simulink model "ENV"  (R2024b)
settings: Solver=FixedStepDiscrete  StartTime=0.0  StopTime=1  FixedStep=0.001  RelTol=1e-3  EnableMultiTasking=on
PreLoadFcn:
  | load('CAN_MESSAGE_bus.mat');
libraries: stm32blockslib x62, canmsglib x28, simulink x6, stm32f4xxblockslib x3
(part 2 of 5)

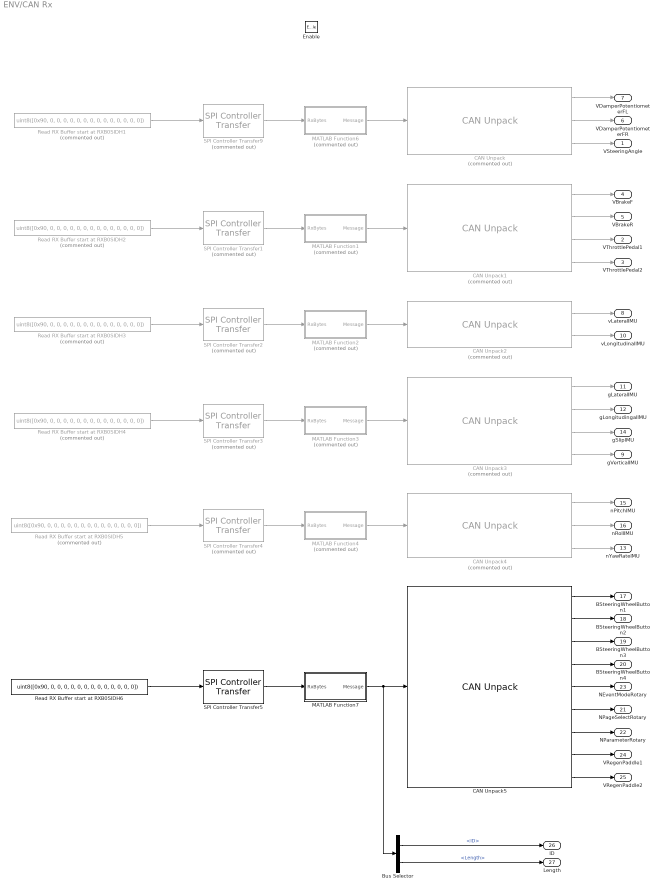
== system ENV/CAN Rx ==
  Enable : EnablePort
  Bus Selector : BusSelector  OutputSignals=ID,Length
  CAN Unpack : canmsglib/CAN Unpack  Commented=on  CANdbFile=C:\Users\oxbro\Documents\STM32CustomProjects\VCUSTM32\OBR26_Controls_30-7-26\CAN\CAN3\CAN3_03.08.26.dbc  MsgList=DDU7_SteerDamper  MsgName=DDU7_SteerDamper  MsgIDType=Standard (11-bit identifier)  MsgIdentifier=257  MsgLength=8  SignalInfo={'VDamperPotentiometerFL','16','13','LE','unsigned','Standard','0','1','0','0','8191';'VDamperPotentiometerFR','29','13','LE','unsigned','Standard','0','1','0','0','8191';'VSteeringAngle','0','13','LE','unsigned','Standard','0','1','0','0','8191'}  IDPort=off  TimestampPort=off  ErrorPort=off  RemotePort=off  LengthPort=off  StatusPort=off  ApplyMinMax=off
      settings: LibrarySourceBlock=stmutilitieslib/CAN Unpack  DataFormat=CANdb specified signals
  CAN Unpack1 : canmsglib/CAN Unpack  Commented=on  CANdbFile=C:\Users\oxbro\Documents\STM32CustomProjects\VCUSTM32\OBR26_Controls_30-7-26\CAN\CAN3\CAN3_03.08.26.dbc  MsgList=DDU7_ThrBrake  MsgName=DDU7_ThrBrake  MsgIDType=Standard (11-bit identifier)  MsgIdentifier=256  MsgLength=8  SignalInfo={'VBrakeF','0','16','LE','unsigned','Standard','0','1','0','0','3276.75';'VBrakeR','16','16','LE','unsigned','Standard','0','1','0','0','65535';'VThrottlePedal1','32','16','LE','unsigned','Standard','0','1','0','0','65535';'VThrottlePedal2','48','16','LE','unsigned','Standard','0','1','0','0','65535'}  IDPort=off  TimestampPort=off  ErrorPort=off  RemotePort=off  LengthPort=off  StatusPort=off  ApplyMinMax=off
      settings: LibrarySourceBlock=stmutilitieslib/CAN Unpack  DataFormat=CANdb specified signals
  CAN Unpack2 : canmsglib/CAN Unpack  Commented=on  CANdbFile=C:\Users\oxbro\Documents\STM32CustomProjects\VCUSTM32\OBR26_Controls_30-7-26\CAN\CAN3\CAN3_03.08.26.dbc  MsgList=IMU_0x604  MsgName=IMU_0x604  MsgIDType=Standard (11-bit identifier)  MsgIdentifier=1540  MsgLength=8  SignalInfo={'vLateralIMU','16','16','LE','signed','Standard','0','0.01','0','-327.68','327.67';'vLongitudinalIMU','0','16','LE','signed','Standard','0','0.01','0','-327.68','327.67'}  IDPort=off  TimestampPort=off  ErrorPort=off  RemotePort=off  LengthPort=off  StatusPort=off  ApplyMinMax=off
      settings: LibrarySourceBlock=stmutilitieslib/CAN Unpack  DataFormat=CANdb specified signals
  CAN Unpack3 : canmsglib/CAN Unpack  Commented=on  CANdbFile=C:\Users\oxbro\Documents\STM32CustomProjects\VCUSTM32\OBR26_Controls_30-7-26\CAN\CAN3\CAN3_03.08.26.dbc  MsgList=IMU_0x606  MsgName=IMU_0x606  MsgIDType=Standard (11-bit identifier)  MsgIdentifier=1542  MsgLength=8  SignalInfo={'gLateralIMU','16','16','LE','signed','Standard','0','0.01','0','-327.68','327.67';'gLongitudinalIMU','0','16','LE','signed','Standard','0','0.01','0','-327.68','327.67';'gSlipIMU','48','16','LE','signed','Standard','0','0.01','0','-327.68','327.67';'gVerticalIMU','32','16','LE','signed','Standard','0','0.01','0','-327.68','327.67'}  IDPort=off  TimestampPort=off  ErrorPort=off  RemotePort=off  LengthPort=off  StatusPort=off  ApplyMinMax=off
      settings: LibrarySourceBlock=stmutilitieslib/CAN Unpack  DataFormat=CANdb specified signals
  CAN Unpack4 : canmsglib/CAN Unpack  Commented=on  CANdbFile=C:\Users\oxbro\Documents\STM32CustomProjects\VCUSTM32\OBR26_Controls_30-7-26\CAN\CAN3\CAN3_03.08.26.dbc  MsgList=IMU_0x609  MsgName=IMU_0x609  MsgIDType=Standard (11-bit identifier)  MsgIdentifier=1545  MsgLength=8  SignalInfo={'nPitchIMU','16','16','LE','signed','Standard','0','0.01','0','-327.68','327.67';'nRollIMU','0','16','LE','signed','Standard','0','0.01','0','-327.68','327.67';'nYawRateIMU','32','16','LE','signed','Standard','0','0.01','0','-327.68','327.67'}  IDPort=off  TimestampPort=off  ErrorPort=off  RemotePort=off  LengthPort=off  StatusPort=off  ApplyMinMax=off
      settings: LibrarySourceBlock=stmutilitieslib/CAN Unpack  DataFormat=CANdb specified signals
  CAN Unpack5 : canmsglib/CAN Unpack  CANdbFile=C:\Users\oxbro\Documents\STM32CustomProjects\VCUSTM32\OBR26_Controls_30-7-26\CAN\CAN3\CAN3_03.08.26.dbc  MsgList=STW_0x1FB  MsgName=STW_0x1FB  MsgIDType=Standard (11-bit identifier)  MsgIdentifier=507  MsgLength=6  SignalInfo={'BSteeringWheelButton1','0','1','LE','unsigned','Standard','0','1','0','0','1';'BSteeringWheelButton2','1','1','LE','unsigned','Standard','0','1','0','0','1';'BSteeringWheelButton3','2','1','LE','unsigned','Standard','0','1','0','0','1';'BSteeringWheelButton4','3','1','LE','unsigned','Standard','0','1','0','0','1';'NEventModeRotary','20','8','LE','unsigned','Standard','0','1','1','1','16';'NPageSelectRotary','4','8','LE','unsigned','Standard','0','1','1','1','16';'NParameterRotary','12','8','LE','unsigned','Standard','0','1','1','1','16';'VRegenPaddle1','28','8','LE','unsigned','Standard','0','0.0129','0','0','3.2895';'VRegenPaddle2','36','8','LE','unsigned','Standard','0','0.0129','0','0','3.2895'}  IDPort=off  TimestampPort=off  ErrorPort=off  RemotePort=off  LengthPort=off  StatusPort=off  ApplyMinMax=off
      settings: LibrarySourceBlock=stmutilitieslib/CAN Unpack  DataFormat=CANdb specified signals
  MATLAB Function1 : MATLAB Function  Commented=on  TreatAsAtomicUnit=on
  MATLAB Function2 : MATLAB Function  Commented=on  TreatAsAtomicUnit=on
  MATLAB Function3 : MATLAB Function  Commented=on  TreatAsAtomicUnit=on
  MATLAB Function4 : MATLAB Function  Commented=on  TreatAsAtomicUnit=on
  MATLAB Function6 : MATLAB Function  Commented=on  TreatAsAtomicUnit=on
  MATLAB Function7 : MATLAB Function  TreatAsAtomicUnit=on
  Read RX Buffer start at RXB0SIDH{1..5} (5 alike) : Constant  Commented=on  Value=uint8([0x90, 0, 0, 0, 0, 0, 0, 0, 0, 0, 0, 0, 0, 0, 0])
  Read RX Buffer start at RXB0SIDH6 : Constant  Value=uint8([0x90, 0, 0, 0, 0, 0, 0, 0, 0, 0, 0, 0, 0, 0])
  SPI Controller Transfer1 : stm32blockslib/SPI Controller Transfer  Priority=2  Commented=on  SPIModuleSelect=SPI1  ClockPolarity=Low  ClockPhase=1 Edge  SPIModule=uint32(0)  Mode=Master  BusSpeed=uint32(1000000)  FirstBitToTransfer=Most significant bit (MSB)  ClockMode=0  BlockFunction=Transfer  EnableRegisterAddress=off  RegisterAddress=0  OutputDataType=uint8  OutputDataLength=1  OutputStatus=off  BlockingMode=on  Timeout=0.01  DataBits=8  UseCustomSSPin=Explicit GPIO calls  ActiveLowSSPin=Active low  Port_Select=GPIOA  Pin=1
      settings: LibrarySourceBlock=stm32h7xxblockslib/SPI Controller Transfer
  SPI Controller Transfer2 : stm32blockslib/SPI Controller Transfer  Priority=3  Commented=on  SPIModuleSelect=SPI1  ClockPolarity=Low  ClockPhase=1 Edge  SPIModule=uint32(0)  Mode=Master  BusSpeed=uint32(1000000)  FirstBitToTransfer=Most significant bit (MSB)  ClockMode=0  BlockFunction=Transfer  EnableRegisterAddress=off  RegisterAddress=0  OutputDataType=uint8  OutputDataLength=1  OutputStatus=off  BlockingMode=on  Timeout=0.01  DataBits=8  UseCustomSSPin=Explicit GPIO calls  ActiveLowSSPin=Active low  Port_Select=GPIOA  Pin=1
      settings: LibrarySourceBlock=stm32h7xxblockslib/SPI Controller Transfer
  SPI Controller Transfer3 : stm32blockslib/SPI Controller Transfer  Priority=4  Commented=on  SPIModuleSelect=SPI1  ClockPolarity=Low  ClockPhase=1 Edge  SPIModule=uint32(0)  Mode=Master  BusSpeed=uint32(1000000)  FirstBitToTransfer=Most significant bit (MSB)  ClockMode=0  BlockFunction=Transfer  EnableRegisterAddress=off  RegisterAddress=0  OutputDataType=uint8  OutputDataLength=1  OutputStatus=off  BlockingMode=on  Timeout=0.01  DataBits=8  UseCustomSSPin=Explicit GPIO calls  ActiveLowSSPin=Active low  Port_Select=GPIOA  Pin=1
      settings: LibrarySourceBlock=stm32h7xxblockslib/SPI Controller Transfer
  SPI Controller Transfer4 : stm32blockslib/SPI Controller Transfer  Priority=5  Commented=on  SPIModuleSelect=SPI1  ClockPolarity=Low  ClockPhase=1 Edge  SPIModule=uint32(0)  Mode=Master  BusSpeed=uint32(1000000)  FirstBitToTransfer=Most significant bit (MSB)  ClockMode=0  BlockFunction=Transfer  EnableRegisterAddress=off  RegisterAddress=0  OutputDataType=uint8  OutputDataLength=1  OutputStatus=off  BlockingMode=on  Timeout=0.01  DataBits=8  UseCustomSSPin=Explicit GPIO calls  ActiveLowSSPin=Active low  Port_Select=GPIOA  Pin=1
      settings: LibrarySourceBlock=stm32h7xxblockslib/SPI Controller Transfer
  SPI Controller Transfer5 : stm32blockslib/SPI Controller Transfer  Priority=6  SPIModuleSelect=SPI1  ClockPolarity=Low  ClockPhase=1 Edge  SPIModule=uint32(0)  Mode=Master  BusSpeed=uint32(1000000)  FirstBitToTransfer=Most significant bit (MSB)  ClockMode=0  BlockFunction=Transfer  EnableRegisterAddress=off  RegisterAddress=0  OutputDataType=uint8  OutputDataLength=1  OutputStatus=off  BlockingMode=on  Timeout=0.01  DataBits=8  UseCustomSSPin=Explicit GPIO calls  ActiveLowSSPin=Active low  Port_Select=GPIOA  Pin=1
      settings: LibrarySourceBlock=stm32h7xxblockslib/SPI Controller Transfer
  SPI Controller Transfer9 : stm32blockslib/SPI Controller Transfer  Priority=1  Commented=on  SPIModuleSelect=SPI1  ClockPolarity=Low  ClockPhase=1 Edge  SPIModule=uint32(0)  Mode=Master  BusSpeed=uint32(1000000)  FirstBitToTransfer=Most significant bit (MSB)  ClockMode=0  BlockFunction=Transfer  EnableRegisterAddress=off  RegisterAddress=0  OutputDataType=uint8  OutputDataLength=1  OutputStatus=off  BlockingMode=on  Timeout=0.01  DataBits=8  UseCustomSSPin=Explicit GPIO calls  ActiveLowSSPin=Active low  Port_Select=GPIOA  Pin=1
      settings: LibrarySourceBlock=stm32h7xxblockslib/SPI Controller Transfer
  VSteeringAngle : Outport  OutDataTypeStr=double
  VThrottlePedal1 : Outport  Port=2  OutDataTypeStr=double
  VThrottlePedal2 : Outport  Port=3  OutDataTypeStr=double
  VBrakeF : Outport  Port=4  OutDataTypeStr=double
  VBrakeR : Outport  Port=5  OutDataTypeStr=double
  VDamperPotentiometerFR : Outport  Port=6  OutDataTypeStr=double
  VDamperPotentiometerFL : Outport  Port=7  OutDataTypeStr=double
  vLateralIMU : Outport  Port=8  OutDataTypeStr=double
  gVerticalIMU : Outport  Port=9  OutDataTypeStr=double
  vLongitudinalIMU : Outport  Port=10  OutDataTypeStr=double
  gLateralIMU : Outport  Port=11  OutDataTypeStr=double
  gLongitudingalIMU : Outport  Port=12  OutDataTypeStr=double
  nYawRateIMU : Outport  Port=13  OutDataTypeStr=double
  gSlipIMU : Outport  Port=14  OutDataTypeStr=double
  nPitchIMU : Outport  Port=15  OutDataTypeStr=double
  nRollIMU : Outport  Port=16  OutDataTypeStr=double
  BSteeringWheelButton1 : Outport  Port=17  OutDataTypeStr=boolean
  BSteeringWheelButton2 : Outport  Port=18  OutDataTypeStr=boolean
  BSteeringWheelButton3 : Outport  Port=19  OutDataTypeStr=boolean
  BSteeringWheelButton4 : Outport  Port=20  OutDataTypeStr=boolean
  NPageSelectRotary : Outport  Port=21  OutDataTypeStr=double
  NParameterRotary : Outport  Port=22  OutDataTypeStr=double
  NEventModeRotary : Outport  Port=23  OutDataTypeStr=double
  VRegenPaddle1 : Outport  Port=24  OutDataTypeStr=double
  VRegenPaddle2 : Outport  Port=25  OutDataTypeStr=double
  ID : Outport  Port=26
  Length : Outport  Port=27
  wires:
  CAN Unpack/1 -> VDamperPotentiometerFL/1
  CAN Unpack/2 -> VDamperPotentiometerFR/1
  CAN Unpack1/2 -> VBrakeR/1
  CAN Unpack1/1 -> VBrakeF/1
  CAN Unpack1/3 -> VThrottlePedal1/1
  CAN Unpack1/4 -> VThrottlePedal2/1
  CAN Unpack/3 -> VSteeringAngle/1
  SPI Controller Transfer9/1 -> MATLAB Function6/1(RxBytes)
  MATLAB Function6/1(Message) -> CAN Unpack/1
  MATLAB Function1/1(Message) -> CAN Unpack1/1
  SPI Controller Transfer1/1 -> MATLAB Function1/1(RxBytes)
  SPI Controller Transfer2/1 -> MATLAB Function2/1(RxBytes)
  MATLAB Function2/1(Message) -> CAN Unpack2/1
  CAN Unpack2/2 -> vLongitudinalIMU/1
  CAN Unpack2/1 -> vLateralIMU/1
  MATLAB Function3/1(Message) -> CAN Unpack3/1
  SPI Controller Transfer3/1 -> MATLAB Function3/1(RxBytes)
  CAN Unpack3/4 -> gVerticalIMU/1
  CAN Unpack3/3 -> gSlipIMU/1
  CAN Unpack3/2 -> gLongitudingalIMU/1
  CAN Unpack3/1 -> gLateralIMU/1
  CAN Unpack4/2 -> nRollIMU/1
  CAN Unpack4/3 -> nYawRateIMU/1
  CAN Unpack4/1 -> nPitchIMU/1
  SPI Controller Transfer4/1 -> MATLAB Function4/1(RxBytes)
  MATLAB Function4/1(Message) -> CAN Unpack4/1
  SPI Controller Transfer5/1 -> MATLAB Function7/1(RxBytes)
  CAN Unpack5/2 -> BSteeringWheelButton2/1
  CAN Unpack5/1 -> BSteeringWheelButton1/1
  CAN Unpack5/3 -> BSteeringWheelButton3/1
  CAN Unpack5/4 -> BSteeringWheelButton4/1
  CAN Unpack5/9 -> VRegenPaddle2/1
  CAN Unpack5/8 -> VRegenPaddle1/1
  CAN Unpack5/7 -> NParameterRotary/1
  CAN Unpack5/6 -> NPageSelectRotary/1
  CAN Unpack5/5 -> NEventModeRotary/1
  Read RX Buffer start at RXB0SIDH1/1 -> SPI Controller Transfer9/1
  Read RX Buffer start at RXB0SIDH6/1 -> SPI Controller Transfer5/1
  Read RX Buffer start at RXB0SIDH5/1 -> SPI Controller Transfer4/1
  Read RX Buffer start at RXB0SIDH4/1 -> SPI Controller Transfer3/1
  Read RX Buffer start at RXB0SIDH3/1 -> SPI Controller Transfer2/1
  Read RX Buffer start at RXB0SIDH2/1 -> SPI Controller Transfer1/1
  MATLAB Function7/1(Message) -> Bus Selector/1, CAN Unpack5/1
  Bus Selector/2 -> Length/1  "<Length>"
  Bus Selector/1 -> ID/1  "<ID>"

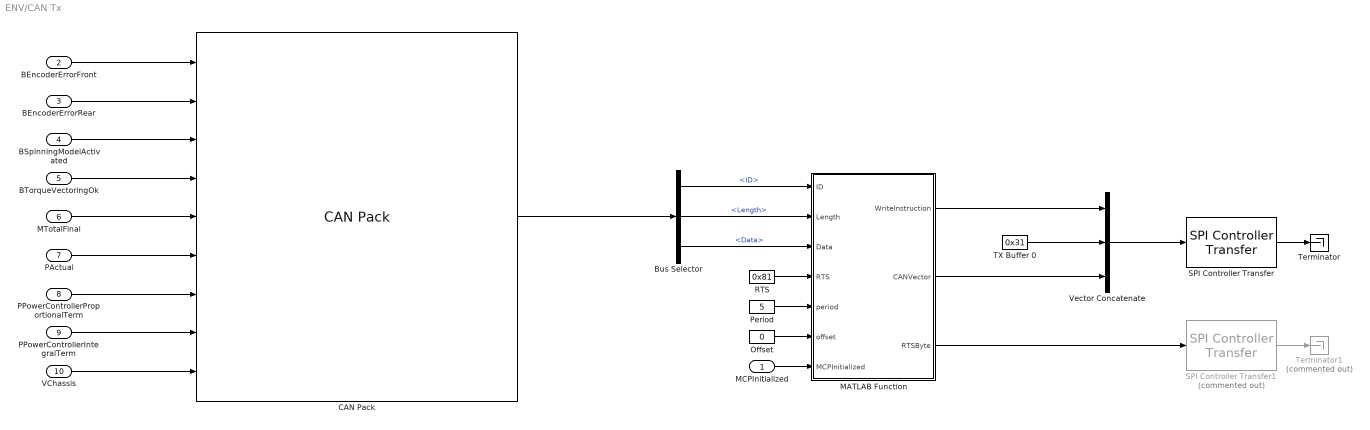
== system ENV/CAN Tx ==
  MCPInitialized : Inport
  BEncoderErrorFront : Inport  Port=2
  BEncoderErrorRear : Inport  Port=3
  BSpinningModelActivated : Inport  Port=4
  BTorqueVectoringOk : Inport  Port=5
  MTotalFinal : Inport  Port=6
  PActual : Inport  Port=7
  PPowerControllerProportionalTerm : Inport  Port=8
  PPowerControllerIntegralTerm : Inport  Port=9
  VChassis : Inport  Port=10
  Bus Selector : BusSelector  OutputSignals=ID,Length,Data
  CAN Pack : canmsglib/CAN Pack  CANdbFile=C:\Users\William\Downloads\VCUSTM32\BaselineControls\CAN\CAN3_baseline.dbc  MsgList=(none)  MsgName=Etas_Signals_01  MsgIDType=Standard (11-bit identifier)  MsgIdentifier=2022  CANIDInput=off  MsgLength=8  Remote=off  ApplyMinMax=off  BusOutput=on  SignalInfo={'BEncoderErrorFront','62','1','LE','unsigned','Standard','0','1','0','0','1';'BEncoderErrorRear','63','1','LE','unsigned','Standard','0','1','0','0','1';'BSpinningModelActivated','60','1','LE','unsigned','Standard','0','1','0','0','1';'BTorqueVectoringOk','61','1','LE','unsigned','Standard','0','1','0','0','1';'MTotalFinal','11','14','LE','signed','Standard','0','0.1','300','-Inf','Inf';'PActual','25','14','LE','signed','Standard','0','0.01','30','-51.92','111.91';'PPowerControlerProportionalTerm','0','11','LE','signed','Standard','0','0.01','0','-10.24','10.23';'PPowerControllerIntergralTerm','49','11','LE','signed','Standard','0','0.01','0','-10.24','10.23';'vChassis','39','10','LE','signed','Standard','0','0.1','0','-51.2','51.1'}
      settings: LibrarySourceBlock=stmutilitieslib/CAN Pack  DataFormat=CANdb specified signals
  MATLAB Function : MATLAB Function  TreatAsAtomicUnit=on
  Offset : Constant  Value=0  OutDataTypeStr=uint16  SampleTime=-1
  Period : Constant  Value=5  OutDataTypeStr=uint16  SampleTime=-1
  RTS : Constant  Value=0x81  OutDataTypeStr=uint8  SampleTime=-1
  SPI Controller Transfer : stm32blockslib/SPI Controller Transfer  Priority=1  SPIModuleSelect=SPI1  ClockPolarity=Low  ClockPhase=1 Edge  SPIModule=uint32(0)  Mode=Master  BusSpeed=uint32(1000000)  FirstBitToTransfer=Most significant bit (MSB)  ClockMode=0  BlockFunction=Transfer  EnableRegisterAddress=off  RegisterAddress=0  OutputDataType=uint8  OutputDataLength=1  OutputStatus=off  BlockingMode=off  Timeout=0.01  DataBits=8  UseCustomSSPin=Explicit GPIO calls  ActiveLowSSPin=Active low  Port_Select=GPIOA  Pin=4
      settings: LibrarySourceBlock=stm32h7xxblockslib/SPI Controller Transfer
  SPI Controller Transfer1 : stm32blockslib/SPI Controller Transfer  Priority=2  Commented=on  SPIModuleSelect=SPI1  ClockPolarity=Low  ClockPhase=1 Edge  SPIModule=uint32(0)  Mode=Master  BusSpeed=uint32(1000000)  FirstBitToTransfer=Most significant bit (MSB)  ClockMode=0  BlockFunction=Transfer  EnableRegisterAddress=off  RegisterAddress=0  OutputDataType=uint8  OutputDataLength=1  OutputStatus=off  BlockingMode=off  Timeout=0.01  DataBits=8  UseCustomSSPin=Explicit GPIO calls  ActiveLowSSPin=Active low  Port_Select=GPIOA  Pin=4
      settings: LibrarySourceBlock=stm32h7xxblockslib/SPI Controller Transfer
  TX Buffer 0 : Constant  Value=0x31  OutDataTypeStr=uint8  SampleTime=-1
  Terminator : Terminator
  Terminator1 : Terminator  Commented=on
  Vector Concatenate : Concatenate  NumInputs=3
  wires:
  CAN Pack/1 -> Bus Selector/1
  BEncoderErrorFront/1 -> CAN Pack/1
  BTorqueVectoringOk/1 -> CAN Pack/4
  BSpinningModelActivated/1 -> CAN Pack/3
  BEncoderErrorRear/1 -> CAN Pack/2
  MTotalFinal/1 -> CAN Pack/5
  PActual/1 -> CAN Pack/6
  PPowerControllerProportionalTerm/1 -> CAN Pack/7
  PPowerControllerIntegralTerm/1 -> CAN Pack/8
  VChassis/1 -> CAN Pack/9
  RTS/1 -> MATLAB Function/4(RTS)
  Bus Selector/1 -> MATLAB Function/1(ID)  "<ID>"
  Bus Selector/2 -> MATLAB Function/2(Length)  "<Length>"
  Bus Selector/3 -> MATLAB Function/3(Data)  "<Data>"
  Offset/1 -> MATLAB Function/6(offset)
  Period/1 -> MATLAB Function/5(period)
  MCPInitialized/1 -> MATLAB Function/7(MCPInitialized)
  Vector Concatenate/1 -> SPI Controller Transfer/1
  MATLAB Function/1(WriteInstruction) -> Vector Concatenate/1
  SPI Controller Transfer1/1 -> Terminator1/1
  TX Buffer 0/1 -> Vector Concatenate/2
  SPI Controller Transfer/1 -> Terminator/1
  MATLAB Function/3(RTSByte) -> SPI Controller Transfer1/1
  MATLAB Function/2(CANVector) -> Vector Concatenate/3

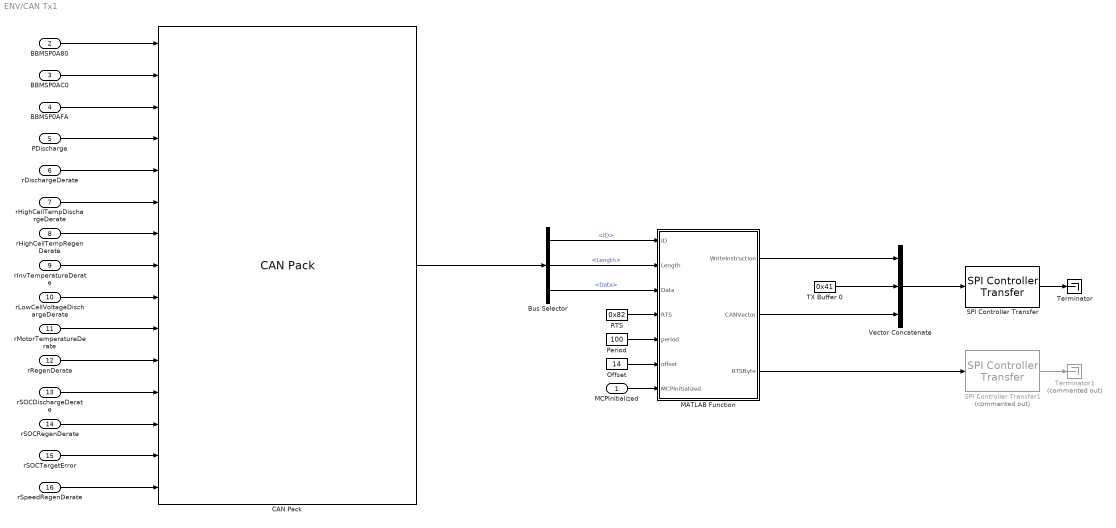
== system ENV/CAN Tx1 ==
  MCPInitialized : Inport
  BBMSP0A80 : Inport  Port=2
  BBMSP0AC0 : Inport  Port=3
  BBMSP0AFA : Inport  Port=4
  PDischarge : Inport  Port=5
  rDischargeDerate : Inport  Port=6
  rHighCellTempDischargeDerate : Inport  Port=7
  rHighCellTempRegenDerate : Inport  Port=8
  rInvTemperatureDerate : Inport  Port=9
  rLowCellVoltageDischargeDerate : Inport  Port=10
  rMotorTemperatureDerate : Inport  Port=11
  rRegenDerate : Inport  Port=12
  rSOCDischargeDerate : Inport  Port=13
  rSOCRegenDerate : Inport  Port=14
  rSOCTargetError : Inport  Port=15
  rSpeedRegenDerate : Inport  Port=16
  Bus Selector : BusSelector  OutputSignals=ID,Length,Data
  CAN Pack : canmsglib/CAN Pack  CANdbFile=C:\Users\William\Downloads\VCUSTM32\BaselineControls\CAN\CAN3_baseline.dbc  MsgList=(none)  MsgName=Etas_Signals_02  MsgIDType=Standard (11-bit identifier)  MsgIdentifier=2023  CANIDInput=off  MsgLength=8  Remote=off  ApplyMinMax=off  BusOutput=on  SignalInfo={'BBMSP0A80','0','1','LE','unsigned','Standard','0','1','0','0','1';'BBMSP0AC0','1','1','LE','unsigned','Standard','0','1','0','0','1';'BBMSP0AFA','2','1','LE','unsigned','Standard','0','1','0','0','1';'PDischarge','43','8','LE','unsigned','Standard','0','1','0','0','255';'rDischargeDerate','35','4','LE','unsigned','Standard','0','0.1','0','0','1.5';'rHighCellTempDischargeDerate','3','4','LE','unsigned','Standard','0','0.1','0','0','1.5';'rHighCellTempRegenDerate','7','4','LE','unsigned','Standard','0','0.1','0','0','1.5';'rInvTemperatureDerate','11','4','LE','unsigned','Standard','0','0.1','0','0','1.5';'rLowCellVoltageDischargeDerate','19','4','LE','unsigned','Standard','0','0.1','0','0','1.5';'rMotorTemperatureDerate','15','4','LE','unsigned','Standard','0','0.1','0','0','1.5';'rRegenDerate','39','4','LE','unsigned','Standard','0','0.1','0','0','1.5';'rSOCDischargeDerate','23','4','LE','unsigned','Standard','0','0.1','0','0','1.5';'rSOCRegenDerate','27','4','LE','unsigned','Standard','0','0.1','0','0','1.5';'rSOCTargetError','51','13','LE','signed','Standard','0','0.001','0','-4.096','4.095';'rSpeedRegenDerate','31','4','LE','unsigned','Standard','0','0.1','0','0','1.5'}
      settings: LibrarySourceBlock=stmutilitieslib/CAN Pack  DataFormat=CANdb specified signals
  MATLAB Function : MATLAB Function  TreatAsAtomicUnit=on
  Offset : Constant  Value=14  OutDataTypeStr=uint16  SampleTime=-1
  Period : Constant  Value=100  OutDataTypeStr=uint16  SampleTime=-1
  RTS : Constant  Value=0x82  OutDataTypeStr=uint8  SampleTime=-1
  SPI Controller Transfer : stm32blockslib/SPI Controller Transfer  Priority=1  SPIModuleSelect=SPI1  ClockPolarity=Low  ClockPhase=1 Edge  SPIModule=uint32(0)  Mode=Master  BusSpeed=uint32(1000000)  FirstBitToTransfer=Most significant bit (MSB)  ClockMode=0  BlockFunction=Transfer  EnableRegisterAddress=off  RegisterAddress=0  OutputDataType=uint8  OutputDataLength=1  OutputStatus=off  BlockingMode=off  Timeout=0.01  DataBits=8  UseCustomSSPin=Explicit GPIO calls  ActiveLowSSPin=Active low  Port_Select=GPIOA  Pin=4
      settings: LibrarySourceBlock=stm32h7xxblockslib/SPI Controller Transfer
  SPI Controller Transfer1 : stm32blockslib/SPI Controller Transfer  Priority=2  Commented=on  SPIModuleSelect=SPI1  ClockPolarity=Low  ClockPhase=1 Edge  SPIModule=uint32(0)  Mode=Master  BusSpeed=uint32(1000000)  FirstBitToTransfer=Most significant bit (MSB)  ClockMode=0  BlockFunction=Transfer  EnableRegisterAddress=off  RegisterAddress=0  OutputDataType=uint8  OutputDataLength=1  OutputStatus=off  BlockingMode=off  Timeout=0.01  DataBits=8  UseCustomSSPin=Explicit GPIO calls  ActiveLowSSPin=Active low  Port_Select=GPIOA  Pin=4
      settings: LibrarySourceBlock=stm32h7xxblockslib/SPI Controller Transfer
  TX Buffer 0 : Constant  Value=0x41  OutDataTypeStr=uint8  SampleTime=-1
  Terminator : Terminator
  Terminator1 : Terminator  Commented=on
  Vector Concatenate : Concatenate  NumInputs=3
  wires:
  BBMSP0AC0/1 -> CAN Pack/2
  BBMSP0A80/1 -> CAN Pack/1
  BBMSP0AFA/1 -> CAN Pack/3
  PDischarge/1 -> CAN Pack/4
  rDischargeDerate/1 -> CAN Pack/5
  rHighCellTempDischargeDerate/1 -> CAN Pack/6
  rHighCellTempRegenDerate/1 -> CAN Pack/7
  rInvTemperatureDerate/1 -> CAN Pack/8
  rLowCellVoltageDischargeDerate/1 -> CAN Pack/9
  rSOCDischargeDerate/1 -> CAN Pack/12
  rSOCRegenDerate/1 -> CAN Pack/13
  rRegenDerate/1 -> CAN Pack/11
  rSOCTargetError/1 -> CAN Pack/14
  rSpeedRegenDerate/1 -> CAN Pack/15
  rMotorTemperatureDerate/1 -> CAN Pack/10
  MATLAB Function/3(RTSByte) -> SPI Controller Transfer1/1
  Bus Selector/3 -> MATLAB Function/3(Data)  "<Data>"
  Offset/1 -> MATLAB Function/6(offset)
  RTS/1 -> MATLAB Function/4(RTS)
  MATLAB Function/1(WriteInstruction) -> Vector Concatenate/1
  Period/1 -> MATLAB Function/5(period)
  Vector Concatenate/1 -> SPI Controller Transfer/1
  Bus Selector/2 -> MATLAB Function/2(Length)  "<Length>"
  SPI Controller Transfer1/1 -> Terminator1/1
  SPI Controller Transfer/1 -> Terminator/1
  TX Buffer 0/1 -> Vector Concatenate/2
  CAN Pack/1 -> Bus Selector/1
  Bus Selector/1 -> MATLAB Function/1(ID)  "<ID>"
  MCPInitialized/1 -> MATLAB Function/7(MCPInitialized)
  MATLAB Function/2(CANVector) -> Vector Concatenate/3

== system ENV/CAN Tx10 ==
  MCPInitialized : Inport
  TEST_NUMBER : Inport  Port=2
  VDamperPotentiometerRL : Inport  Port=3
  VDamperPotentiometerRR : Inport  Port=4
  Bus Selector : BusSelector  OutputSignals=ID,Length,Data
  CAN Pack : canmsglib/CAN Pack  CANdbFile=C:\Users\William\Downloads\VCUSTM32\BaselineControls\CAN\CAN3_baseline.dbc  MsgList=(none)  MsgName=Etas_Signals_11  MsgIDType=Standard (11-bit identifier)  MsgIdentifier=1796  CANIDInput=off  MsgLength=6  Remote=off  ApplyMinMax=off  BusOutput=on  SignalInfo={'TEST_NUMBER','32','16','LE','unsigned','Standard','0','1','0','-32768','32767';'VDamperPotentiometerRL','0','10','LE','unsigned','Standard','0','0.005','0','0','5.115';'VDamperPotentiometerRR','16','10','LE','unsigned','Standard','0','0.005','0','0','5.115'}
      settings: LibrarySourceBlock=stmutilitieslib/CAN Pack  DataFormat=CANdb specified signals
  MATLAB Function : MATLAB Function  TreatAsAtomicUnit=on
  Offset : Constant  Value=8  OutDataTypeStr=uint16  SampleTime=-1
  Period : Constant  Value=100  OutDataTypeStr=uint16  SampleTime=-1
  RTS : Constant  Value=0x82  OutDataTypeStr=uint8  SampleTime=-1
  SPI Controller Transfer : stm32blockslib/SPI Controller Transfer  Priority=1  SPIModuleSelect=SPI1  ClockPolarity=Low  ClockPhase=1 Edge  SPIModule=uint32(0)  Mode=Master  BusSpeed=uint32(1000000)  FirstBitToTransfer=Most significant bit (MSB)  ClockMode=0  BlockFunction=Transfer  EnableRegisterAddress=off  RegisterAddress=0  OutputDataType=uint8  OutputDataLength=1  OutputStatus=off  BlockingMode=off  Timeout=0.01  DataBits=8  UseCustomSSPin=Explicit GPIO calls  ActiveLowSSPin=Active low  Port_Select=GPIOA  Pin=4
      settings: LibrarySourceBlock=stm32h7xxblockslib/SPI Controller Transfer
  SPI Controller Transfer1 : stm32blockslib/SPI Controller Transfer  Priority=2  Commented=on  SPIModuleSelect=SPI1  ClockPolarity=Low  ClockPhase=1 Edge  SPIModule=uint32(0)  Mode=Master  BusSpeed=uint32(1000000)  FirstBitToTransfer=Most significant bit (MSB)  ClockMode=0  BlockFunction=Transfer  EnableRegisterAddress=off  RegisterAddress=0  OutputDataType=uint8  OutputDataLength=1  OutputStatus=off  BlockingMode=off  Timeout=0.01  DataBits=8  UseCustomSSPin=Explicit GPIO calls  ActiveLowSSPin=Active low  Port_Select=GPIOA  Pin=4
      settings: LibrarySourceBlock=stm32h7xxblockslib/SPI Controller Transfer
  TX Buffer 0 : Constant  Value=0x41  OutDataTypeStr=uint8  SampleTime=-1
  Terminator : Terminator
  Terminator1 : Terminator  Commented=on
  Vector Concatenate : Concatenate  NumInputs=3
  wires:
  VDamperPotentiometerRL/1 -> CAN Pack/2
  TEST_NUMBER/1 -> CAN Pack/1
  RTS/1 -> MATLAB Function/4(RTS)
  MATLAB Function/1(WriteInstruction) -> Vector Concatenate/1
  TX Buffer 0/1 -> Vector Concatenate/2
  SPI Controller Transfer1/1 -> Terminator1/1
  MATLAB Function/2(CANVector) -> Vector Concatenate/3
  Offset/1 -> MATLAB Function/6(offset)
  Bus Selector/2 -> MATLAB Function/2(Length)  "<Length>"
  Bus Selector/3 -> MATLAB Function/3(Data)  "<Data>"
  Vector Concatenate/1 -> SPI Controller Transfer/1
  MCPInitialized/1 -> MATLAB Function/7(MCPInitialized)
  Period/1 -> MATLAB Function/5(period)
  Bus Selector/1 -> MATLAB Function/1(ID)  "<ID>"
  CAN Pack/1 -> Bus Selector/1
  SPI Controller Transfer/1 -> Terminator/1
  MATLAB Function/3(RTSByte) -> SPI Controller Transfer1/1
  VDamperPotentiometerRR/1 -> CAN Pack/3

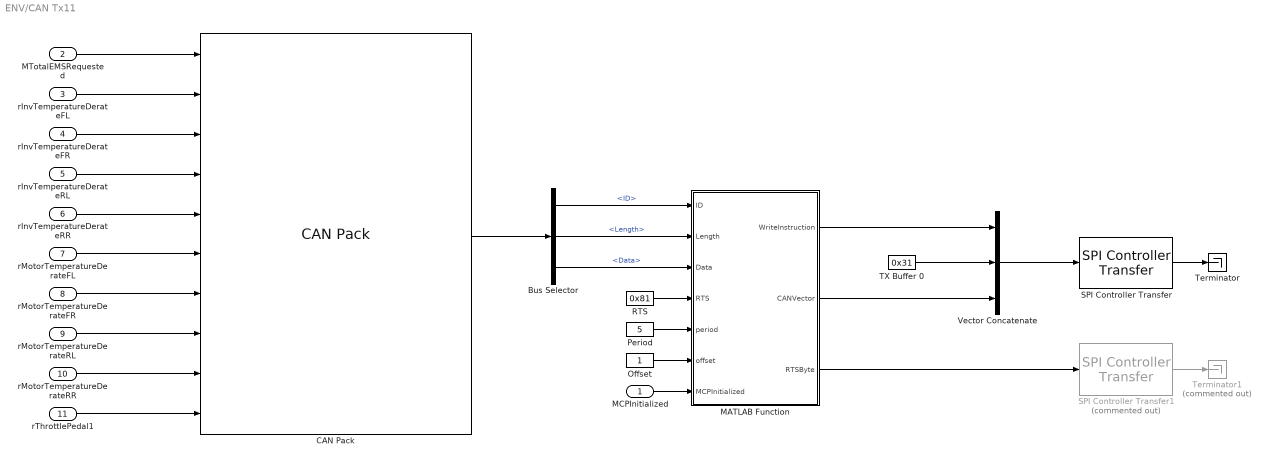
== system ENV/CAN Tx11 ==
  MCPInitialized : Inport
  MTotalEMSRequested : Inport  Port=2
  rInvTemperatureDerateFL : Inport  Port=3
  rInvTemperatureDerateFR : Inport  Port=4
  rInvTemperatureDerateRL : Inport  Port=5
  rInvTemperatureDerateRR : Inport  Port=6
  rMotorTemperatureDerateFL : Inport  Port=7
  rMotorTemperatureDerateFR : Inport  Port=8
  rMotorTemperatureDerateRL : Inport  Port=9
  rMotorTemperatureDerateRR : Inport  Port=10
  rThrottlePedal1 : Inport  Port=11
  Bus Selector : BusSelector  OutputSignals=ID,Length,Data
  CAN Pack : canmsglib/CAN Pack  CANdbFile=C:\Users\William\Downloads\VCUSTM32\BaselineControls\CAN\CAN3_baseline.dbc  MsgList=(none)  MsgName=Etas_Signals_12  MsgIDType=Standard (11-bit identifier)  MsgIdentifier=2039  CANIDInput=off  MsgLength=8  Remote=off  ApplyMinMax=off  BusOutput=on  SignalInfo={'MTotalEMSRequested','32','14','LE','signed','Standard','0','0.1','300','-519.2','1119.1';'rInvTemperatureDerateFL','4','4','LE','unsigned','Standard','0','0.1','0','0','1.5';'rInvTemperatureDerateFR','8','4','LE','unsigned','Standard','0','0.1','0','0','1.5';'rInvTemperatureDerateRL','12','4','LE','unsigned','Standard','0','0.1','0','0','1.5';'rInvTemperatureDerateRR','16','4','LE','unsigned','Standard','0','0.1','0','0','1.5';'rMotorTemperatureDerateFL','20','4','LE','unsigned','Standard','0','0.1','0','0','1.5';'rMotorTemperatureDerateFR','24','4','LE','unsigned','Standard','0','0.1','0','0','1.5';'rMotorTemperatureDerateRL','28','4','LE','unsigned','Standard','0','0.1','0','-Inf','Inf';'rMotorTemperatureDerateRR','0','4','LE','unsigned','Standard','0','0.1','0','0','1.5';'rThrottlePedal1','46','10','LE','unsigned','Standard','0','0.1','0','0','102.3'}
      settings: LibrarySourceBlock=stmutilitieslib/CAN Pack  DataFormat=CANdb specified signals
  MATLAB Function : MATLAB Function  TreatAsAtomicUnit=on
  Offset : Constant  OutDataTypeStr=uint16  SampleTime=-1
  Period : Constant  Value=5  OutDataTypeStr=uint16  SampleTime=-1
  RTS : Constant  Value=0x81  OutDataTypeStr=uint8  SampleTime=-1
  SPI Controller Transfer : stm32blockslib/SPI Controller Transfer  Priority=1  SPIModuleSelect=SPI1  ClockPolarity=Low  ClockPhase=1 Edge  SPIModule=uint32(0)  Mode=Master  BusSpeed=uint32(1000000)  FirstBitToTransfer=Most significant bit (MSB)  ClockMode=0  BlockFunction=Transfer  EnableRegisterAddress=off  RegisterAddress=0  OutputDataType=uint8  OutputDataLength=1  OutputStatus=off  BlockingMode=off  Timeout=0.01  DataBits=8  UseCustomSSPin=Explicit GPIO calls  ActiveLowSSPin=Active low  Port_Select=GPIOA  Pin=4
      settings: LibrarySourceBlock=stm32h7xxblockslib/SPI Controller Transfer
  SPI Controller Transfer1 : stm32blockslib/SPI Controller Transfer  Priority=2  Commented=on  SPIModuleSelect=SPI1  ClockPolarity=Low  ClockPhase=1 Edge  SPIModule=uint32(0)  Mode=Master  BusSpeed=uint32(1000000)  FirstBitToTransfer=Most significant bit (MSB)  ClockMode=0  BlockFunction=Transfer  EnableRegisterAddress=off  RegisterAddress=0  OutputDataType=uint8  OutputDataLength=1  OutputStatus=off  BlockingMode=off  Timeout=0.01  DataBits=8  UseCustomSSPin=Explicit GPIO calls  ActiveLowSSPin=Active low  Port_Select=GPIOA  Pin=4
      settings: LibrarySourceBlock=stm32h7xxblockslib/SPI Controller Transfer
  TX Buffer 0 : Constant  Value=0x31  OutDataTypeStr=uint8  SampleTime=-1
  Terminator : Terminator
  Terminator1 : Terminator  Commented=on
  Vector Concatenate : Concatenate  NumInputs=3
  wires:
  rInvTemperatureDerateFL/1 -> CAN Pack/2
  MTotalEMSRequested/1 -> CAN Pack/1
  rInvTemperatureDerateFR/1 -> CAN Pack/3
  rInvTemperatureDerateRL/1 -> CAN Pack/4
  rInvTemperatureDerateRR/1 -> CAN Pack/5
  rMotorTemperatureDerateFL/1 -> CAN Pack/6
  rMotorTemperatureDerateFR/1 -> CAN Pack/7
  rMotorTemperatureDerateRL/1 -> CAN Pack/8
  rMotorTemperatureDerateRR/1 -> CAN Pack/9
  rThrottlePedal1/1 -> CAN Pack/10
  RTS/1 -> MATLAB Function/4(RTS)
  MATLAB Function/1(WriteInstruction) -> Vector Concatenate/1
  TX Buffer 0/1 -> Vector Concatenate/2
  SPI Controller Transfer1/1 -> Terminator1/1
  MATLAB Function/2(CANVector) -> Vector Concatenate/3
  Offset/1 -> MATLAB Function/6(offset)
  Bus Selector/2 -> MATLAB Function/2(Length)  "<Length>"
  Bus Selector/3 -> MATLAB Function/3(Data)  "<Data>"
  Vector Concatenate/1 -> SPI Controller Transfer/1
  MCPInitialized/1 -> MATLAB Function/7(MCPInitialized)
  Period/1 -> MATLAB Function/5(period)
  Bus Selector/1 -> MATLAB Function/1(ID)  "<ID>"
  CAN Pack/1 -> Bus Selector/1
  SPI Controller Transfer/1 -> Terminator/1
  MATLAB Function/3(RTSByte) -> SPI Controller Transfer1/1

== system ENV/CAN Tx12 ==
  MCPInitialized : Inport
  nMotorFL : Inport  Port=2
  nMotorFR : Inport  Port=3
  nMotorRL : Inport  Port=4
  nMotorRR : Inport  Port=5
  Bus Selector : BusSelector  OutputSignals=ID,Length,Data
  CAN Pack : canmsglib/CAN Pack  CANdbFile=C:\Users\William\Downloads\VCUSTM32\BaselineControls\CAN\CAN3_baseline.dbc  MsgList=(none)  MsgName=Etas_Signals_13  MsgIDType=Standard (11-bit identifier)  MsgIdentifier=2008  CANIDInput=off  MsgLength=8  Remote=off  ApplyMinMax=off  BusOutput=on  SignalInfo={'nMotorFL','0','16','LE','signed','Standard','0','1','0','-32768','32767';'nMotorFR','16','16','LE','signed','Standard','0','1','0','-32768','32767';'nMotorRL','32','16','LE','signed','Standard','0','1','0','-32768','32767';'nMotorRR','48','16','LE','signed','Standard','0','1','0','-32768','32767'}
      settings: LibrarySourceBlock=stmutilitieslib/CAN Pack  DataFormat=CANdb specified signals
  MATLAB Function : MATLAB Function  TreatAsAtomicUnit=on
  Offset : Constant  OutDataTypeStr=uint16  SampleTime=-1
  Period : Constant  Value=10  OutDataTypeStr=uint16  SampleTime=-1
  RTS : Constant  Value=0x82  OutDataTypeStr=uint8  SampleTime=-1
  SPI Controller Transfer : stm32blockslib/SPI Controller Transfer  Priority=1  SPIModuleSelect=SPI1  ClockPolarity=Low  ClockPhase=1 Edge  SPIModule=uint32(0)  Mode=Master  BusSpeed=uint32(1000000)  FirstBitToTransfer=Most significant bit (MSB)  ClockMode=0  BlockFunction=Transfer  EnableRegisterAddress=off  RegisterAddress=0  OutputDataType=uint8  OutputDataLength=1  OutputStatus=off  BlockingMode=off  Timeout=0.01  DataBits=8  UseCustomSSPin=Explicit GPIO calls  ActiveLowSSPin=Active low  Port_Select=GPIOA  Pin=4
      settings: LibrarySourceBlock=stm32h7xxblockslib/SPI Controller Transfer
  SPI Controller Transfer1 : stm32blockslib/SPI Controller Transfer  Priority=2  Commented=on  SPIModuleSelect=SPI1  ClockPolarity=Low  ClockPhase=1 Edge  SPIModule=uint32(0)  Mode=Master  BusSpeed=uint32(1000000)  FirstBitToTransfer=Most significant bit (MSB)  ClockMode=0  BlockFunction=Transfer  EnableRegisterAddress=off  RegisterAddress=0  OutputDataType=uint8  OutputDataLength=1  OutputStatus=off  BlockingMode=off  Timeout=0.01  DataBits=8  UseCustomSSPin=Explicit GPIO calls  ActiveLowSSPin=Active low  Port_Select=GPIOA  Pin=4
      settings: LibrarySourceBlock=stm32h7xxblockslib/SPI Controller Transfer
  TX Buffer 0 : Constant  Value=0x41  OutDataTypeStr=uint8  SampleTime=-1
  Terminator : Terminator
  Terminator1 : Terminator  Commented=on
  Vector Concatenate : Concatenate  NumInputs=3
  wires:
  nMotorFR/1 -> CAN Pack/2
  nMotorFL/1 -> CAN Pack/1
  nMotorRL/1 -> CAN Pack/3
  nMotorRR/1 -> CAN Pack/4
  Bus Selector/2 -> MATLAB Function/2(Length)  "<Length>"
  Vector Concatenate/1 -> SPI Controller Transfer/1
  Bus Selector/1 -> MATLAB Function/1(ID)  "<ID>"
  SPI Controller Transfer/1 -> Terminator/1
  Period/1 -> MATLAB Function/5(period)
  MATLAB Function/1(WriteInstruction) -> Vector Concatenate/1
  MATLAB Function/3(RTSByte) -> SPI Controller Transfer1/1
  RTS/1 -> MATLAB Function/4(RTS)
  SPI Controller Transfer1/1 -> Terminator1/1
  Bus Selector/3 -> MATLAB Function/3(Data)  "<Data>"
  Offset/1 -> MATLAB Function/6(offset)
  MATLAB Function/2(CANVector) -> Vector Concatenate/3
  CAN Pack/1 -> Bus Selector/1
  TX Buffer 0/1 -> Vector Concatenate/2
  MCPInitialized/1 -> MATLAB Function/7(MCPInitialized)

== system ENV/CAN Tx13 ==
  MCPInitialized : Inport
  BDischargeAllowed : Inport  Port=2
  BEMS1000mPoint : Inport  Port=3
  BEMS995mPoint : Inport  Port=4
  MDriverDischargeRequested : Inport  Port=5
  MFLFinal : Inport  Port=6
  MFRFinal : Inport  Port=7
  MRLFinal : Inport  Port=8
  MRRFinal : Inport  Port=9
  Bus Selector : BusSelector  OutputSignals=ID,Length,Data
  CAN Pack : canmsglib/CAN Pack  CANdbFile=C:\Users\William\Downloads\VCUSTM32\BaselineControls\CAN\CAN3_baseline.dbc  MsgList=(none)  MsgName=Etas_Signals_14  MsgIDType=Standard (11-bit identifier)  MsgIdentifier=2009  CANIDInput=off  MsgLength=8  Remote=off  ApplyMinMax=off  BusOutput=on  SignalInfo={'BDischargeAllowed','63','1','LE','unsigned','Standard','0','1','0','0','1';'BEMS1000mPoint','61','1','LE','unsigned','Standard','0','1','0','0','1';'BEMS995mPoint','62','1','LE','unsigned','Standard','0','1','0','0','1';'MDriverDischargeRequested','48','13','LE','unsigned','Standard','0','0.1','0','0','819.1';'MFLFinal','12','12','LE','signed','Standard','0','0.1','50','-154.8','254.7';'MFRFinal','0','12','LE','signed','Standard','0','0.1','50','-154.8','254.7';'MRLFinal','24','12','LE','signed','Standard','0','0.1','50','-154.8','254.7';'MRRFinal','36','12','LE','signed','Standard','0','0.1','50','-154.8','254.7'}
      settings: LibrarySourceBlock=stmutilitieslib/CAN Pack  DataFormat=CANdb specified signals
  MATLAB Function : MATLAB Function  TreatAsAtomicUnit=on
  Offset : Constant  Value=2  OutDataTypeStr=uint16  SampleTime=-1
  Period : Constant  Value=5  OutDataTypeStr=uint16  SampleTime=-1
  RTS : Constant  Value=0x81  OutDataTypeStr=uint8  SampleTime=-1
  SPI Controller Transfer : stm32blockslib/SPI Controller Transfer  Priority=1  SPIModuleSelect=SPI1  ClockPolarity=Low  ClockPhase=1 Edge  SPIModule=uint32(0)  Mode=Master  BusSpeed=uint32(1000000)  FirstBitToTransfer=Most significant bit (MSB)  ClockMode=0  BlockFunction=Transfer  EnableRegisterAddress=off  RegisterAddress=0  OutputDataType=uint8  OutputDataLength=1  OutputStatus=off  BlockingMode=off  Timeout=0.01  DataBits=8  UseCustomSSPin=Explicit GPIO calls  ActiveLowSSPin=Active low  Port_Select=GPIOA  Pin=4
      settings: LibrarySourceBlock=stm32h7xxblockslib/SPI Controller Transfer
  SPI Controller Transfer1 : stm32blockslib/SPI Controller Transfer  Priority=2  Commented=on  SPIModuleSelect=SPI1  ClockPolarity=Low  ClockPhase=1 Edge  SPIModule=uint32(0)  Mode=Master  BusSpeed=uint32(1000000)  FirstBitToTransfer=Most significant bit (MSB)  ClockMode=0  BlockFunction=Transfer  EnableRegisterAddress=off  RegisterAddress=0  OutputDataType=uint8  OutputDataLength=1  OutputStatus=off  BlockingMode=off  Timeout=0.01  DataBits=8  UseCustomSSPin=Explicit GPIO calls  ActiveLowSSPin=Active low  Port_Select=GPIOA  Pin=4
      settings: LibrarySourceBlock=stm32h7xxblockslib/SPI Controller Transfer
  TX Buffer 0 : Constant  Value=0x31  OutDataTypeStr=uint8  SampleTime=-1
  Terminator : Terminator
  Terminator1 : Terminator  Commented=on
  Vector Concatenate : Concatenate  NumInputs=3
  wires:
  BEMS1000mPoint/1 -> CAN Pack/2
  BDischargeAllowed/1 -> CAN Pack/1
  BEMS995mPoint/1 -> CAN Pack/3
  MDriverDischargeRequested/1 -> CAN Pack/4
  MFLFinal/1 -> CAN Pack/5
  MFRFinal/1 -> CAN Pack/6
  MRLFinal/1 -> CAN Pack/7
  MRRFinal/1 -> CAN Pack/8
  CAN Pack/1 -> Bus Selector/1
  SPI Controller Transfer/1 -> Terminator/1
  Bus Selector/1 -> MATLAB Function/1(ID)  "<ID>"
  Period/1 -> MATLAB Function/5(period)
  Bus Selector/3 -> MATLAB Function/3(Data)  "<Data>"
  Vector Concatenate/1 -> SPI Controller Transfer/1
  Bus Selector/2 -> MATLAB Function/2(Length)  "<Length>"
  Offset/1 -> MATLAB Function/6(offset)
  SPI Controller Transfer1/1 -> Terminator1/1
  MATLAB Function/2(CANVector) -> Vector Concatenate/3
  TX Buffer 0/1 -> Vector Concatenate/2
  MATLAB Function/3(RTSByte) -> SPI Controller Transfer1/1
  RTS/1 -> MATLAB Function/4(RTS)
  MCPInitialized/1 -> MATLAB Function/7(MCPInitialized)
  MATLAB Function/1(WriteInstruction) -> Vector Concatenate/1

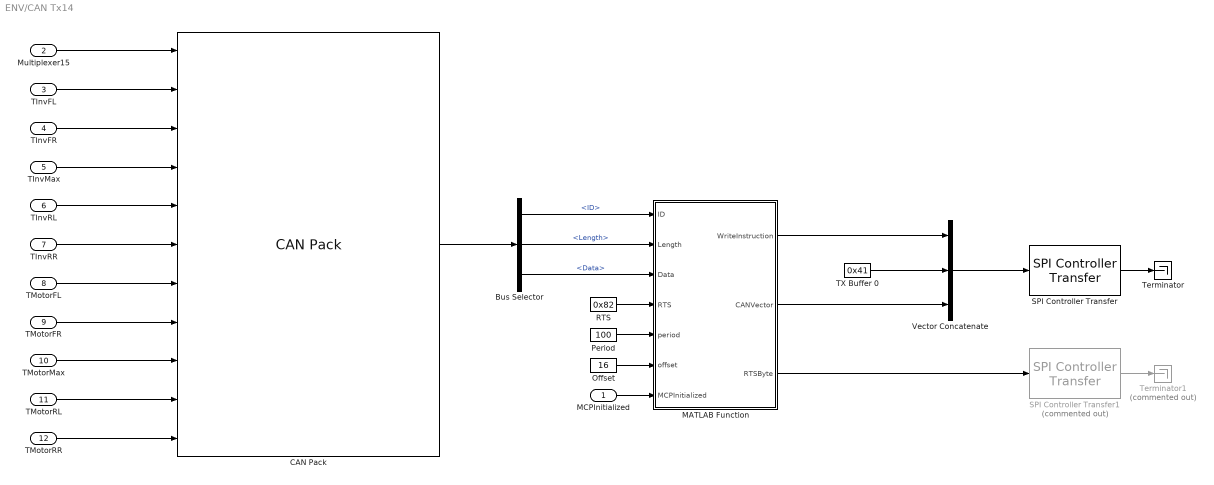
== system ENV/CAN Tx14 ==
  MCPInitialized : Inport
  Multiplexer15 : Inport  Port=2
  TInvFL : Inport  Port=3
  TInvFR : Inport  Port=4
  TInvMax : Inport  Port=5
  TInvRL : Inport  Port=6
  TInvRR : Inport  Port=7
  TMotorFL : Inport  Port=8
  TMotorFR : Inport  Port=9
  TMotorMax : Inport  Port=10
  TMotorRL : Inport  Port=11
  TMotorRR : Inport  Port=12
  Bus Selector : BusSelector  OutputSignals=ID,Length,Data
  CAN Pack : canmsglib/CAN Pack  CANdbFile=C:\Users\William\Downloads\VCUSTM32\BaselineControls\CAN\CAN3_baseline.dbc  MsgList=(none)  MsgName=Etas_Signals_15  MsgIDType=Standard (11-bit identifier)  MsgIdentifier=2017  CANIDInput=off  MsgLength=8  Remote=off  ApplyMinMax=off  BusOutput=on  SignalInfo={'Multiplexer15','62','2','LE','unsigned','Multiplexor','0','1','0','0','3';'TInvFL','10','10','LE','unsigned','Multiplexed','1','0.1','0','0','102.3';'TInvFR','20','10','LE','unsigned','Multiplexed','1','0.1','0','0','102.3';'TInvMax','30','10','LE','unsigned','Multiplexed','1','0.1','0','0','102.3';'TInvRL','40','10','LE','unsigned','Multiplexed','1','0.1','0','0','102.3';'TInvRR','0','10','LE','unsigned','Multiplexed','1','0.1','0','0','102.3';'TMotorFL','12','11','LE','unsigned','Multiplexed','0','0.1','0','0','204.7';'TMotorFR','0','11','LE','unsigned','Multiplexed','0','0.1','0','0','204.7';'TMotorMax','45','11','LE','unsigned','Multiplexed','0','0.1','0','0','204.7';'TMotorRL','23','11','LE','unsigned','Multiplexed','0','0.1','0','0','204.7';'TMotorRR','34','11','LE','unsigned','Multiplexed','0','0.1','0','0','204.7'}
      settings: LibrarySourceBlock=stmutilitieslib/CAN Pack  DataFormat=CANdb specified signals
  MATLAB Function : MATLAB Function  TreatAsAtomicUnit=on
  Offset : Constant  Value=16  OutDataTypeStr=uint16  SampleTime=-1
  Period : Constant  Value=100  OutDataTypeStr=uint16  SampleTime=-1
  RTS : Constant  Value=0x82  OutDataTypeStr=uint8  SampleTime=-1
  SPI Controller Transfer : stm32blockslib/SPI Controller Transfer  Priority=1  SPIModuleSelect=SPI1  ClockPolarity=Low  ClockPhase=1 Edge  SPIModule=uint32(0)  Mode=Master  BusSpeed=uint32(1000000)  FirstBitToTransfer=Most significant bit (MSB)  ClockMode=0  BlockFunction=Transfer  EnableRegisterAddress=off  RegisterAddress=0  OutputDataType=uint8  OutputDataLength=1  OutputStatus=off  BlockingMode=off  Timeout=0.01  DataBits=8  UseCustomSSPin=Explicit GPIO calls  ActiveLowSSPin=Active low  Port_Select=GPIOA  Pin=4
      settings: LibrarySourceBlock=stm32h7xxblockslib/SPI Controller Transfer
  SPI Controller Transfer1 : stm32blockslib/SPI Controller Transfer  Priority=2  Commented=on  SPIModuleSelect=SPI1  ClockPolarity=Low  ClockPhase=1 Edge  SPIModule=uint32(0)  Mode=Master  BusSpeed=uint32(1000000)  FirstBitToTransfer=Most significant bit (MSB)  ClockMode=0  BlockFunction=Transfer  EnableRegisterAddress=off  RegisterAddress=0  OutputDataType=uint8  OutputDataLength=1  OutputStatus=off  BlockingMode=off  Timeout=0.01  DataBits=8  UseCustomSSPin=Explicit GPIO calls  ActiveLowSSPin=Active low  Port_Select=GPIOA  Pin=4
      settings: LibrarySourceBlock=stm32h7xxblockslib/SPI Controller Transfer
  TX Buffer 0 : Constant  Value=0x41  OutDataTypeStr=uint8  SampleTime=-1
  Terminator : Terminator
  Terminator1 : Terminator  Commented=on
  Vector Concatenate : Concatenate  NumInputs=3
  wires:
  TInvFL/1 -> CAN Pack/2
  Multiplexer15/1 -> CAN Pack/1
  TInvFR/1 -> CAN Pack/3
  TInvMax/1 -> CAN Pack/4
  TInvRL/1 -> CAN Pack/5
  TInvRR/1 -> CAN Pack/6
  TMotorFL/1 -> CAN Pack/7
  TMotorFR/1 -> CAN Pack/8
  TMotorMax/1 -> CAN Pack/9
  TMotorRL/1 -> CAN Pack/10
  TMotorRR/1 -> CAN Pack/11
  CAN Pack/1 -> Bus Selector/1
  SPI Controller Transfer/1 -> Terminator/1
  Bus Selector/1 -> MATLAB Function/1(ID)  "<ID>"
  Period/1 -> MATLAB Function/5(period)
  Bus Selector/3 -> MATLAB Function/3(Data)  "<Data>"
  Vector Concatenate/1 -> SPI Controller Transfer/1
  Bus Selector/2 -> MATLAB Function/2(Length)  "<Length>"
  Offset/1 -> MATLAB Function/6(offset)
  SPI Controller Transfer1/1 -> Terminator1/1
  MATLAB Function/2(CANVector) -> Vector Concatenate/3
  TX Buffer 0/1 -> Vector Concatenate/2
  MATLAB Function/3(RTSByte) -> SPI Controller Transfer1/1
  RTS/1 -> MATLAB Function/4(RTS)
  MCPInitialized/1 -> MATLAB Function/7(MCPInitialized)
  MATLAB Function/1(WriteInstruction) -> Vector Concatenate/1

== system ENV/CAN Tx15 ==
  MCPInitialized : Inport
  NInvDTCFL : Inport  Port=2
  NInvDTCFR : Inport  Port=3
  NInvDTCRL : Inport  Port=4
  NInvDTCRR : Inport  Port=5
  TCellMax : Inport  Port=6
  VCellDelta : Inport  Port=7
  Bus Selector : BusSelector  OutputSignals=ID,Length,Data
  CAN Pack : canmsglib/CAN Pack  CANdbFile=C:\Users\William\Downloads\VCUSTM32\BaselineControls\CAN\CAN3_baseline.dbc  MsgList=(none)  MsgName=Etas_Signals_16  MsgIDType=Standard (11-bit identifier)  MsgIdentifier=2018  CANIDInput=off  MsgLength=8  Remote=off  ApplyMinMax=off  BusOutput=on  SignalInfo={'NInvDTCFL','12','12','LE','unsigned','Standard','0','1','0','0','4095';'NInvDTCFR','24','12','LE','unsigned','Standard','0','1','0','0','4095';'NinvDTCRL','36','12','LE','unsigned','Standard','0','1','0','0','4095';'NinvDTCRR','0','12','LE','unsigned','Standard','0','1','0','0','4095';'TCellMax','48','10','LE','unsigned','Standard','0','0.1','0','0','102.3';'VCellDelta','58','6','LE','unsigned','Standard','0','0.01','0','0','0.63'}
      settings: LibrarySourceBlock=stmutilitieslib/CAN Pack  DataFormat=CANdb specified signals
  MATLAB Function : MATLAB Function  TreatAsAtomicUnit=on
  Offset : Constant  Value=3  OutDataTypeStr=uint16  SampleTime=-1
  Period : Constant  Value=5  OutDataTypeStr=uint16  SampleTime=-1
  RTS : Constant  Value=0x81  OutDataTypeStr=uint8  SampleTime=-1
  SPI Controller Transfer : stm32blockslib/SPI Controller Transfer  Priority=1  SPIModuleSelect=SPI1  ClockPolarity=Low  ClockPhase=1 Edge  SPIModule=uint32(0)  Mode=Master  BusSpeed=uint32(1000000)  FirstBitToTransfer=Most significant bit (MSB)  ClockMode=0  BlockFunction=Transfer  EnableRegisterAddress=off  RegisterAddress=0  OutputDataType=uint8  OutputDataLength=1  OutputStatus=off  BlockingMode=off  Timeout=0.01  DataBits=8  UseCustomSSPin=Explicit GPIO calls  ActiveLowSSPin=Active low  Port_Select=GPIOA  Pin=4
      settings: LibrarySourceBlock=stm32h7xxblockslib/SPI Controller Transfer
  SPI Controller Transfer1 : stm32blockslib/SPI Controller Transfer  Priority=2  Commented=on  SPIModuleSelect=SPI1  ClockPolarity=Low  ClockPhase=1 Edge  SPIModule=uint32(0)  Mode=Master  BusSpeed=uint32(1000000)  FirstBitToTransfer=Most significant bit (MSB)  ClockMode=0  BlockFunction=Transfer  EnableRegisterAddress=off  RegisterAddress=0  OutputDataType=uint8  OutputDataLength=1  OutputStatus=off  BlockingMode=off  Timeout=0.01  DataBits=8  UseCustomSSPin=Explicit GPIO calls  ActiveLowSSPin=Active low  Port_Select=GPIOA  Pin=4
      settings: LibrarySourceBlock=stm32h7xxblockslib/SPI Controller Transfer
  TX Buffer 0 : Constant  Value=0x31  OutDataTypeStr=uint8  SampleTime=-1
  Terminator : Terminator
  Terminator1 : Terminator  Commented=on
  Vector Concatenate : Concatenate  NumInputs=3
  wires:
  NInvDTCFR/1 -> CAN Pack/2
  NInvDTCFL/1 -> CAN Pack/1
  NInvDTCRL/1 -> CAN Pack/3
  NInvDTCRR/1 -> CAN Pack/4
  TCellMax/1 -> CAN Pack/5
  VCellDelta/1 -> CAN Pack/6
  Bus Selector/2 -> MATLAB Function/2(Length)  "<Length>"
  MCPInitialized/1 -> MATLAB Function/7(MCPInitialized)
  Vector Concatenate/1 -> SPI Controller Transfer/1
  Bus Selector/3 -> MATLAB Function/3(Data)  "<Data>"
  Offset/1 -> MATLAB Function/6(offset)
  MATLAB Function/3(RTSByte) -> SPI Controller Transfer1/1
  Period/1 -> MATLAB Function/5(period)
  MATLAB Function/2(CANVector) -> Vector Concatenate/3
  Bus Selector/1 -> MATLAB Function/1(ID)  "<ID>"
  SPI Controller Transfer1/1 -> Terminator1/1
  SPI Controller Transfer/1 -> Terminator/1
  TX Buffer 0/1 -> Vector Concatenate/2
  MATLAB Function/1(WriteInstruction) -> Vector Concatenate/1
  RTS/1 -> MATLAB Function/4(RTS)
  CAN Pack/1 -> Bus Selector/1
